simulink model "untitled1"  (R2018b)
settings: Solver=VariableStepAuto  StartTime=0.0  StopTime=10.0  RelTol=1e-3
settings Model: Creator=a4327  LastModifiedBy=a4327

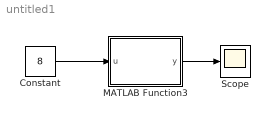
== system untitled1 ==
  Constant : Constant  Value=8
  MATLAB Function3 : MATLAB Function  TreatAsAtomicUnit=on
  Scope : Scope
  wires:
  Constant/1 -> MATLAB Function3/1(u)
  MATLAB Function3/1(y) -> Scope/1

== matlab function untitled1/MATLAB Function3 ==
  data: u input; y output
function y = wrap_PI(u)
y = wrap_PI(u);
